simulink model "HardMon_Diego"  (R2023b)
settings: Solver=FixedStepDiscrete  StartTime=0.0  StopTime=10.0  FixedStep=0.1  RelTol=1e-3  EnableMultiTasking=on
settings Model: Creator=diego  LastModifiedBy=diego
settings SolverCC: AlgebraicLoopSolver=TrustRegion  AutoInsertRateTranBlk=on
settings DataIOCC: LimitDataPoints=on
settings OptimizationCC: LifeSpan=inf
settings DebuggingCC: UnconnectedInputMsg=warning  UnconnectedOutputMsg=warning  UnconnectedLineMsg=warning  AllowSymbolicDim=off  SFUnexpectedBacktrackingDiag=warning  SFNoUnconditionalDefaultTransitionDiag=warning  SFExecutionAtInitializationDiag=none  ArithmeticOperatorsInVariantConditions=warning
settings ModelReferenceCC: EnableRefExpFcnMdlSchedulingChecks=on
settings SFSimCC: SimUseLocalCustomCode=off  CustomCodeUndefinedFunction=UseInterfaceOnly
settings RTWCC: RTWUseLocalCustomCode=off  DLArmComputeVersion=19.05
settings CodeAppCC: StateflowObjectComments=on
settings GRTTargetCC: TargetLangStandard=C89/C90 (ANSI)
settings ConfigComp: CovMetricSettings=dw  CovSaveCumulativeToWorkspaceVar=on  CovSaveSingleToWorkspaceVar=on  CovExternalEMLEnable=off  CovSFcnEnable=off

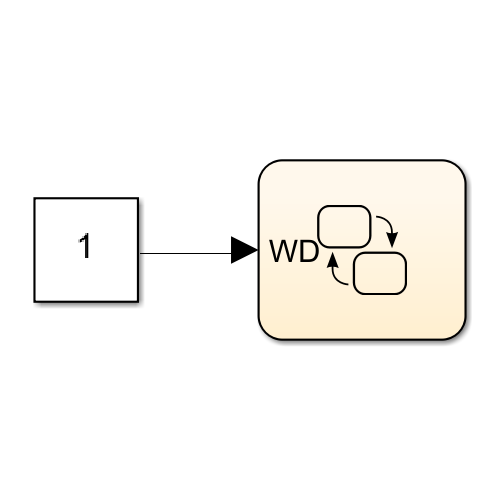
[thumbnail: Simulink's stored preview of the top-level diagram]
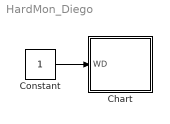
== system HardMon_Diego ==
  Chart : Stateflow chart  TreatAsAtomicUnit=on
  Constant : Constant
  wires:
  Constant/1 -> Chart/1(WD)

== stateflow chart HardMon_Diego/Chart ==
  state Normal
    entry:
    WD_Copy = WD;
    state after
      (default) -> (junction 12) : % if
      (junction 12) -> (junction 13) [order 1] : [WD_Copy == WD]
      (junction 12) -> (junction 14) [order 2]
      (junction 13) -> (junction 15) : {fault = 1;}
      (junction 15) -> (junction 14)
      (junction 14) -> (junction 16)
    state Default
    (default) -> Default
    Default -> after : after(4,sec)
  state Fault
  (default) -> Normal
  Normal -> Fault : [fault == 1]
  data: WD_Copy local; WD input; fault local =0
